simulink model "HardwareValidation_HWTest_2024_Proper"  (R2024b)
settings: Solver=ode1  StartTime=0.0  StopTime=inf  FixedStep=0.002  RelTol=1e-3  EnableMultiTasking=on
PostLoadFcn:
  | qc_set_target_type(getConfigSet(bdroot, 'QUARC Default Target Configuration'));
undefined symbols (not defined in the file): A_obs_hw, B_obs_hw, C_obs_hw, D_obs_hw, HIL, hw_use_augmented_controller, hw_use_observer, K_aug_hw, K_hw, V_sat
libraries: quarc_library x4
settings Model: SimulationMode=external  ExtModeTrigDuration=5000  Creator=pmartin  LastModifiedBy=Student
settings SolverCC: AlgebraicLoopSolver=TrustRegion  PositivePriorityOrder=on
settings DataIOCC: LimitDataPoints=on  SaveFormat=Array  SignalLoggingSaveFormat=ModelDataLogs  ReturnWorkspaceOutputs=off
settings OptimizationCC: ExpressionDepthLimit=2147483647  InitFltsAndDblsToZero=on
settings DebuggingCC: SaveWithParameterizedLinksMsg=none  UnderspecifiedInitializationDetection=Classic  MergeDetectMultiDrivingBlocksExec=none  SolverPrmCheckMsg=warning  MultiTaskDSMMsg=warning  MultiTaskCondExecSysMsg=none  FcnCallInpInsideContextMsg=warning  UnconnectedInputMsg=warning  UnconnectedOutputMsg=warning  UnconnectedLineMsg=warning  StateNameClashWarn=warning  SFUnexpectedBacktrackingDiag=warning  SFNoUnconditionalDefaultTransitionDiag=warning  SFExecutionAtInitializationDiag=none  ArithmeticOperatorsInVariantConditions=warning
settings ModelReferenceCC: PropagateSignalLabelsOutOfModel=off
settings SFSimCC: SimUseLocalCustomCode=off  CustomCodeUndefinedFunction=UseInterfaceOnly
settings RTWCC: Description=QUARC Win64 Target Using Toolchain  SystemTargetFile=quarc_win64.tlc  TemplateMakefile=quarc_default_tmf  RTWUseLocalCustomCode=off  Toolchain=QUARC win64 | nmake (64-bit Windows)  BuildConfiguration=Faster Runs  GPUComputeCapability=3.5
settings CodeAppCC: StateflowObjectComments=on
settings STFCustomTargetCC: ConcurrentExecutionCompliant=on  GRTInterface=on  UseToolchainInfoCompliant=on  SystemTargetFile=quarc_win64.tlc
settings GRTTargetCC: TargetLangStandard=C89/C90 (ANSI)  ParMdlRefBuildCompliant=off  CompOptLevelCompliant=off  CombineOutputUpdateFcns=off  MatFileLogging=off  CPPClassGenCompliant=off  GRTInterface=on  ExtMode=on  ExtModeMexFile=quarc_comm
settings ConfigComp: CovMetricSettings=dw  CovSaveCumulativeToWorkspaceVar=on  CovSaveSingleToWorkspaceVar=on  CovExternalEMLEnable=off

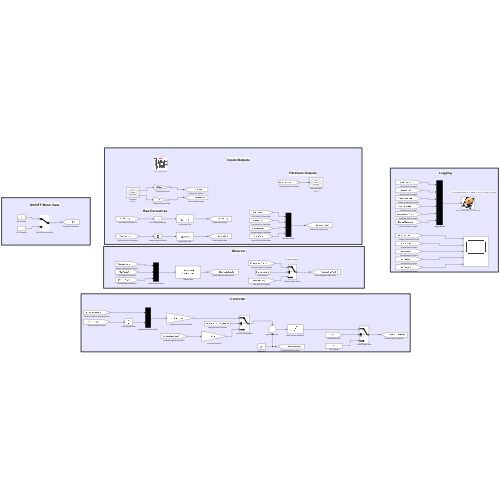
[thumbnail: Simulink's stored preview of the top-level diagram]
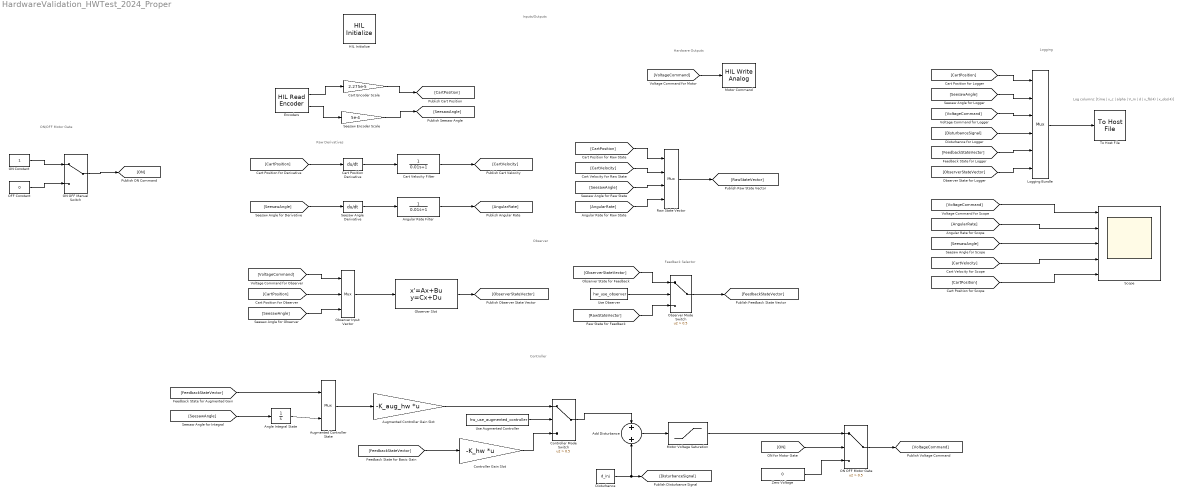
== system HardwareValidation_HWTest_2024_Proper ==
  note: Log columns: [time | x_c | alpha | V_m | d | x_fb(4) | x_obs(4)]
  note: Observer
  note: Logging
  note: Hardware Outputs
  note: Inputs/Outputs
  note: Controller
  note: Raw Derivatives
  note: ON/OFF Motor Gate
  note: Feedback Selector
  Add Disturbance : Sum
  Angle Integral State : Integrator
  Angular Rate Filter : TransferFcn  Denominator=[0.01 1]
  Augmented Controller Gain Slot : Gain  Gain=-K_aug_hw  Multiplication=Matrix(K*u)
  Augmented Controller State : Mux  Inputs=2
  Cart Encoder Scale : Gain  Gain=2.275e-5
  Cart Position Derivative : Derivative
  Cart Velocity Filter : TransferFcn  Denominator=[0.01 1]
  Controller Gain Slot : Gain  Gain=-K_hw  Multiplication=Matrix(K*u)
  Controller Mode Switch : Switch  Criteria=u2 > Threshold  Threshold=0.5  SaturateOnIntegerOverflow=off  InputSameDT=off
  Disturbance : FromWorkspace  VariableName=d_inj
  Encoders : quarc_library/Data Acquisition/Generic/Immediate I//O/HIL Read Encoder  object_name=HIL-1  channels=[0:1]  sample_time=qc_get_step_size  active=on  vector_output=off  data_type_mode=Inherit via back propagation  data_type=double
  HIL Initialize : quarc_library/Data Acquisition/Generic/Configuration/HIL Initialize  object_name=HIL-1  board_type=q2_usb  board_number=0  board_options=d0=digital;d1=digital;led=auto;update_rate=normal  exclusive=off  active=off  hardware_clocks=[0:2]  clock_modes=[]  initial_clock_frequencies=[]  set_clock_params_at_start=off  set_clock_params_at_switch_in=off  set_clock_frequencies_at_start=off  set_clock_frequencies_at_switch_in=off  analog_input_channels=[0:1]  analog_input_configurations=[]  analog_input_maximums=10  analog_input_minimums=-10  set_analog_input_params_at_start=on  set_analog_input_params_at_switch_in=off  analog_output_channels=[0:1]  analog_output_maximums=10  analog_output_minimums=-10  initial_analog_outputs=[0]  final_analog_outputs=[0]  watchdog_analog_outputs=0  set_analog_output_params_at_start=on  set_analog_output_params_at_switch_in=off  set_analog_outputs_at_start=on  set_analog_outputs_at_switch_in=off  set_analog_outputs_at_terminate=on  set_analog_outputs_at_switch_out=off  set_analog_outputs_on_watchdog=off  digital_input_channels=[]  digital_output_channels=[0:7]  digital_output_configuration=[]  initial_digital_outputs=[0]  final_digital_outputs=[0]  watchdog_digital_outputs=[0]  set_digital_output_params_at_start=off  set_digital_output_params_at_switch_in=off  set_digital_outputs_at_start=on  set_digital_outputs_at_switch_in=off  set_digital_outputs_at_terminate=on  set_digital_outputs_at_switch_out=off  set_digital_outputs_on_watchdog=off  encoder_channels=[0:1]  quadrature=[4]  encoder_filter_frequency=[]  initial_encoder_counts=[0]  set_encoder_params_at_start=on  set_encoder_params_at_switch_in=off  set_encoder_counts_at_start=on  set_encoder_counts_at_switch_in=off  pwm_channels=[]  pwm_modes=[0]  pwm_frequency=1/0.020  pwm_configuration=[]  pwm_alignment=[]  pwm_polarity=[]  pwm_leading_deadband=[]  pwm_trailing_deadband=[]  initial_pwm_outputs=[0]  final_pwm_outputs=[0]  watchdog_pwm_outputs=[0]  set_pwm_params_at_start=on  set_pwm_params_at_switch_in=off  set_pwm_outputs_at_start=on  set_pwm_outputs_at_switch_in=off  set_pwm_outputs_at_terminate=on  set_pwm_outputs_at_switch_out=off  set_pwm_outputs_on_watchdog=off  other_output_channels=[]  initial_other_outputs=[]  final_other_outputs=[]  watchdog_other_outputs=[]  set_other_outputs_at_start=off  set_other_outputs_at_switch_in=off  set_other_outputs_at_terminate=off  set_other_outputs_at_switch_out=off  set_other_outputs_on_watchdog=off
  Logging Bundle : Mux  Inputs=6
  Motor Command : quarc_library/Data Acquisition/Generic/Immediate I//O/HIL Write Analog  object_name=HIL-1  channels=0  sample_time=-1  active=off  vector_input=off
  Motor Voltage Saturation : Saturate  UpperLimit=V_sat  LowerLimit=-V_sat
  OFF Constant : Constant  Value=0
  ON Constant : Constant
  ON OFF Manual Switch : ManualSwitch
  ON OFF Motor Gate : Switch  Criteria=u2 > Threshold  Threshold=0.5  SaturateOnIntegerOverflow=off  InputSameDT=off
  Observer Input Vector : Mux  Inputs=3
  Observer Mode Switch : Switch  Criteria=u2 > Threshold  Threshold=0.5  SaturateOnIntegerOverflow=off  InputSameDT=off
  Observer Slot : StateSpace  A=A_obs_hw  B=B_obs_hw  C=C_obs_hw  D=D_obs_hw  InitialCondition=[0; 0; 0; 0]
  Raw State Vector : Mux
  Scope : Scope  NumInputPorts=5
  Seesaw Angle Derivative : Derivative
  Seesaw Encoder Scale : Gain  Gain=5e-4
  To Host File : quarc_library/Sinks/To Host/To Host File  source=Specify via dialog (do not evaluate)  file_name=data_%{date}_%{time}.mat  variable_name=data  decimation=1  sample_time=-1  file_format=MAT-file v.4  options=No header or footer  append=off  final_file_name=data_19-May-2026_17-00-41.mat  encoding=Default  bitrate=0
  Use Augmented Controller : Constant  Value=hw_use_augmented_controller
  Use Observer : Constant  Value=hw_use_observer
  Zero Voltage : Constant  Value=0
  wires:
  Disturbance/1 -> [DisturbanceSignal], Add Disturbance/2
  [CartVelocity] -> Raw State Vector/2
  [SeesawAngle] -> Logging Bundle/2
  Angular Rate Filter/1 -> [AngularRate]
  [FeedbackStateVector] -> Controller Gain Slot/1
  Augmented Controller State/1 -> Augmented Controller Gain Slot/1
  Cart Encoder Scale/1 -> [CartPosition]
  Use Augmented Controller/1 -> Controller Mode Switch/2
  Angle Integral State/1 -> Augmented Controller State/2
  Motor Voltage Saturation/1 -> ON OFF Motor Gate/1
  Observer Input Vector/1 -> Observer Slot/1
  Encoders/1 -> Cart Encoder Scale/1
  [VoltageCommand] -> Logging Bundle/3
  [SeesawAngle] -> Angle Integral State/1
  [CartPosition] -> Raw State Vector/1
  [CartPosition] -> Logging Bundle/1
  Augmented Controller Gain Slot/1 -> Controller Mode Switch/1
  Logging Bundle/1 -> To Host File/1
  OFF Constant/1 -> ON OFF Manual Switch/2
  Add Disturbance/1 -> Motor Voltage Saturation/1
  [SeesawAngle] -> Raw State Vector/3
  ON Constant/1 -> ON OFF Manual Switch/1
  [DisturbanceSignal] -> Logging Bundle/4
  Encoders/2 -> Seesaw Encoder Scale/1
  [CartPosition] -> Scope/5
  ON OFF Motor Gate/1 -> [VoltageCommand]
  [VoltageCommand] -> Scope/1
  [AngularRate] -> Raw State Vector/4
  [CartVelocity] -> Scope/4
  Raw State Vector/1 -> [RawStateVector]
  Observer Mode Switch/1 -> [FeedbackStateVector]
  [ObserverStateVector] -> Logging Bundle/6
  [CartPosition] -> Observer Input Vector/2
  Cart Position Derivative/1 -> Cart Velocity Filter/1
  Seesaw Encoder Scale/1 -> [SeesawAngle]
  [SeesawAngle] -> Scope/3
  [VoltageCommand] -> Observer Input Vector/1
  [ObserverStateVector] -> Observer Mode Switch/1
  [VoltageCommand] -> Motor Command/1
  [AngularRate] -> Scope/2
  [FeedbackStateVector] -> Augmented Controller State/1
  Observer Slot/1 -> [ObserverStateVector]
  [SeesawAngle] -> Seesaw Angle Derivative/1
  Zero Voltage/1 -> ON OFF Motor Gate/3
  [FeedbackStateVector] -> Logging Bundle/5
  Use Observer/1 -> Observer Mode Switch/2
  [CartPosition] -> Cart Position Derivative/1
  [RawStateVector] -> Observer Mode Switch/3
  [SeesawAngle] -> Observer Input Vector/3
  Controller Mode Switch/1 -> Add Disturbance/1
  Cart Velocity Filter/1 -> [CartVelocity]
  Seesaw Angle Derivative/1 -> Angular Rate Filter/1
  ON OFF Manual Switch/1 -> [ON]
  [ON] -> ON OFF Motor Gate/2
  Controller Gain Slot/1 -> Controller Mode Switch/3
